simulink library "findDotCentroidPosition_ul"  (R2018b)
settings: Solver=VariableStepAuto  StartTime=0.0  StopTime=10.0  RelTol=1e-3
values from neighbouring files (symbols this model uses):
  camPositionVec_cm = [0 0 0]    [findDotCentroidPosition_ts.m]
undefined symbols (not defined in the file or in its folder): camFOVVec_deg
settings Model: Creator=mcobb  LastModifiedBy=mcobb
settings DebuggingCC: LibraryContextMissingDiagnostic=none
settings SFSimCC: SimUseLocalCustomCode=off
settings RTWCC: RTWUseLocalCustomCode=off

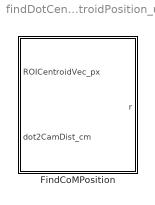
== system findDotCentroidPosition_ul ==
  FindCoMPosition : Subsystem  mask{camPositionVec_cm=camPositionVec_cm, cameraViewAngleVec_deg=camFOVVec_deg, cam2GroundRotationMatrix=0, imageDimensions_px=0}
      mask prompts: camPositionVec_cm "Camera Position Vector [cm]"; cameraViewAngleVec_deg "Camera View Angle [horizontal vertical] [deg]"; cam2GroundRotationMatrix "Camera Rotation Matrix"; imageDimensions_px "Image Dimensions [rows cols]"

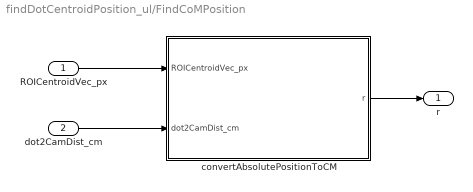
== system findDotCentroidPosition_ul/FindCoMPosition ==
  ROICentroidVec_px : Inport  PortDimensions=2
  dot2CamDist_cm : Inport  Port=2  PortDimensions=1
  convertAbsolutePositionToCM : MATLAB Function  TreatAsAtomicUnit=on
  r : Outport
  wires:
  convertAbsolutePositionToCM/1(r) -> r/1
  ROICentroidVec_px/1 -> convertAbsolutePositionToCM/1(ROICentroidVec_px)
  dot2CamDist_cm/1 -> convertAbsolutePositionToCM/2(dot2CamDist_cm)

== matlab function findDotCentroidPosition_ul/FindCoMPosition/convertAbsolutePositionToCM ==
  data: ROICentroidVec_px input; dot2CamDist_cm input; r output size=3; camPositionVec_cm parameter; cam2GroundRotationMatrix parameter; imageDimensions_px parameter; cameraViewAngleVec_deg parameter
function r = convertAbsolutePositionsToCM(ROICentroidVec_px,dot2CamDist_cm,...
    camPositionVec_cm, cam2GroundRotationMatrix, imageDimensions_px,...
    cameraViewAngleVec_deg)
%#codegen
% This function calculates the x, y and z position of the dots in the
% ground fixed coordinates

% INPUTS
% rCam - 3 element vector of the camera position in the ground fixed frame
% units:cm
% xCam - horitontal location of the dots centroid in the image frame
% units:pixels
% yCam - vertical location of the dots centroid in the image frame
% units:pixels
% viewAngle - two element vector, first characterizes the width of the
% field of view (camera horizontal), the second characterizes the height of
% the field of veiw (camera vertical).
% d - distance from the camera to the dots

% Calculate the x and y locations
% If the horizontal location of the dots centroid in the image frame is
% to the left of the centerline (xCam<1020) then the y position of the dots
% centroid in the ground fixed frame will be less than the y position of
% the camera in the ground fixed frame.
% If the vertical location of the dots centroid in the image frame is
% below the centerline (yCam>544) then the x position of the dots
% centroid in the ground fixed frame will be greater than the x position of
% the camera in the ground fixed frame.
% d=50;

% x = rCam(1) + (yCam - 544 )*((2*d*tand(viewAngle(1)))/1088);
% y = rCam(2) + (xCam - 1020)*((2*d*tand(viewAngle(2)))/2040);
%
% % Calculate the z coordinate of the centroid of the dots.
% % We know the x and y coordinate, the position of the camera, and the
% % distance fromt the cammera to the dots.  Therfore, the solution is the
% % value of z which causes the position to lie on the sphere centered on the
% % camera with radius = d
% z = 0;
% % Check first to make sure that the value under the sqrt is positive
% if d^2-(x - rCam(1))^2-(y - rCam(2))^2>=0
%     z  = rCam(3) + sqrt(d^2-(x - rCam(1))^2-(y - rCam(2))^2);
% end
%
% r  =  [x y z];

%% New code starts here

% Calculate the x and y position in the camera frame
% x = rCam(1) + (yCam - 544 )*((2*d*tand(viewAngle(1)))/1088);
% y = rCam(2) + (xCam - 1020)*((2*d*tand(viewAngle(2)))/2040);

x = (ROICentroidVec_px(1) - imageDimensions_px(1)/2 )*...
    ((2*dot2CamDist_cm*tand(cameraViewAngleVec_deg(1)))/imageDimensions_px(1));

y = (ROICentroidVec_px(2) - imageDimensions_px(2)/2 )*...
    ((2*dot2CamDist_cm*tand(cameraViewAngleVec_deg(2)))/imageDimensions_px(2));

% Calculate z based on the known distance from the camera to the dot
% centroid
z = 0;
if dot2CamDist_cm^2-x^2-y^2>=0
    z = -sqrt(dot2CamDist_cm^2-x^2-y^2);
end
% r = zeros(3,1);


r = cam2GroundRotationMatrix*[x y z]' + reshape(camPositionVec_cm,[],1);
r(abs(r)<10e-10)=0;
% r = [0 0 0];
